simulink model "ResistiveLoad"  (R2019a)
settings: Solver=VariableStepAuto  StartTime=0.0  StopTime=2  RelTol=1e-3
libraries: powerlib x16, powerlib_meascontrol x2, simulink x1
settings Model: Creator=hakan  LastModifiedBy=hakan

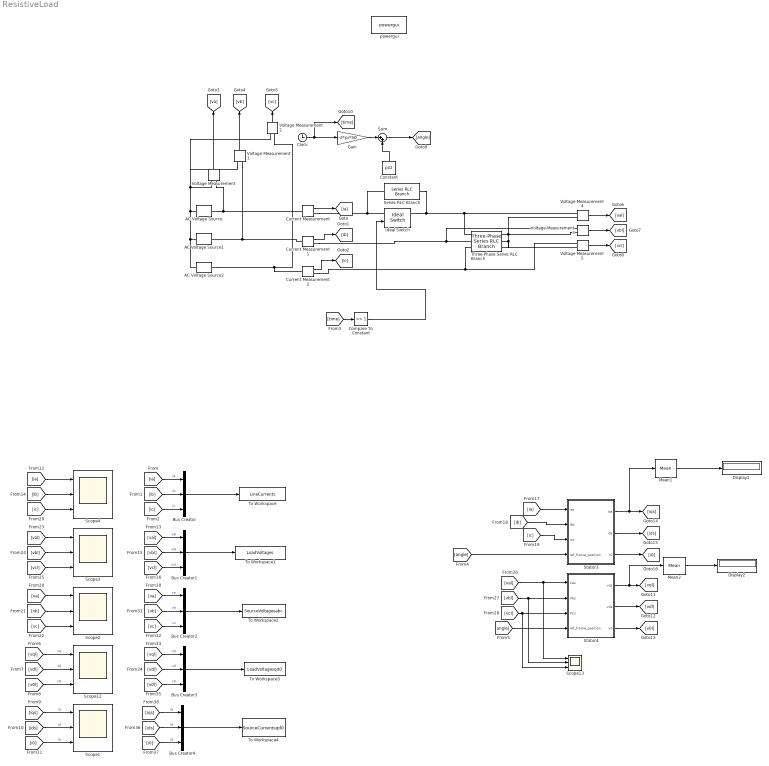
== system ResistiveLoad ==
  AC Voltage Source : powerlib/Electrical Sources/AC Voltage Source  Amplitude=400  Phase=0  Frequency=50  SampleTime=0  Measurements=None  BusType=swing  Pref=10e3  Qref=0  Qmin=-inf  Qmax=+inf
      settings: SourceProductName=Simscape Electrical
  AC Voltage Source1 : powerlib/Electrical Sources/AC Voltage Source  Amplitude=400  Phase=120  Frequency=50  SampleTime=0  Measurements=None  BusType=swing  Pref=10e3  Qref=0  Qmin=-inf  Qmax=+inf
      settings: SourceProductName=Simscape Electrical
  AC Voltage Source2 : powerlib/Electrical Sources/AC Voltage Source  Amplitude=400  Phase=240  Frequency=50  SampleTime=0  Measurements=None  BusType=swing  Pref=10e3  Qref=0  Qmin=-inf  Qmax=+inf
      settings: SourceProductName=Simscape Electrical
  Bus Creator{,1..4} (5 alike) : BusCreator  Inputs=3
  Clock : Clock
  Compare To Constant : simulink/Logic and Bit Operations/Compare To Constant  relop=<=  const=1  OutDataTypeStr=boolean
  Constant : Constant  Value=pi/2
  Current Measurement : powerlib/Measurements/Current Measurement  PhasorSimulation=off  OutputType=Complex  PSBequivalent=0
      settings: SourceProductName=Simscape Electrical
  Current Measurement1 : powerlib/Measurements/Current Measurement  PhasorSimulation=off  OutputType=Complex  PSBequivalent=0
      settings: SourceProductName=Simscape Electrical
  Current Measurement2 : powerlib/Measurements/Current Measurement  PhasorSimulation=off  OutputType=Complex  PSBequivalent=0
      settings: SourceProductName=Simscape Electrical
  Display1 : Display
      settings: Decimation=5
  Display2 : Display
      settings: Decimation=5
  Gain : Gain  Gain=-2*pi*50
  Ideal Switch : powerlib/Power Electronics/Ideal Switch  Ron=0.001  Lon=0  IC=0  Rs=1e5  Cs=inf  Measurements=on
      settings: SourceProductName=Simscape Electrical
  Mean1 : powerlib_meascontrol/Measurements/Mean  Freq=25  Vinit=0  Ts=0
      settings: SourceProductName=Simscape Electrical
  Mean2 : powerlib_meascontrol/Measurements/Mean  Freq=25  Vinit=0  Ts=0
      settings: SourceProductName=Simscape Electrical
  Scope{1..4,12..13} (6 alike) : Scope  NumInputPorts=3
  Series RLC Branch : powerlib/Elements/Series RLC Branch  LConnTagsString=__new0  RConnTagsString=__new0  BranchType=R  Resistance=500000000000  Inductance=1e-3  SetiL0=off  InitialCurrent=0  Capacitance=1e-6  Setx0=off  InitialVoltage=0  Measurements=None
      settings: SourceProductName=Simscape Electrical
  Stator3 : MATLAB Function  TreatAsAtomicUnit=on
  Stator4 : MATLAB Function  TreatAsAtomicUnit=on
  Sum : Sum  Inputs=|++
  Three-Phase Series RLC Branch : powerlib/Elements/Three-Phase Series RLC Branch  LConnTagsString=A|B|C  RConnTagsString=A|B|C  BranchType=R  Resistance=1  Inductance=1e-3  Capacitance=1e-6  Measurements=None
      settings: SourceProductName=Simscape Electrical
  To Workspace : ToWorkspace  VariableName=LineCurrents  SaveFormat=Timeseries  SampleTime=-1
  To Workspace1 : ToWorkspace  VariableName=LoadVoltages  SaveFormat=Timeseries  SampleTime=-1
  To Workspace2 : ToWorkspace  VariableName=SourceVoltagesabc  SaveFormat=Timeseries  SampleTime=-1
  To Workspace3 : ToWorkspace  VariableName=LoadVoltagesqd0  SaveFormat=Timeseries  SampleTime=-1
  To Workspace4 : ToWorkspace  VariableName=SourceCurrentsqd0  SaveFormat=Timeseries  SampleTime=-1
  Voltage Measurement{,1..5} (6 alike) : powerlib/Measurements/Voltage Measurement  PhasorSimulation=off  OutputType=Complex  PSBequivalent=0
      settings: SourceProductName=Simscape Electrical
  powergui : powerlib/powergui  Priority=1  SimulationMode=Discrete  SampleTime=10e-6  frequency=60  Iterations=50  frequencyindice=50  Pbase=100e6  ErrMax=1e-4  UnitsV=kV  UnitsW=MW  buscounter=0  FunctionMessages=off  echomessages=off  EnableUseOfTLC=off  CurrentSourceSwitches=off  DisableSnubberDevices=off  DisableRonSwitches=off  DisableVfSwitches=off  DisplayEquations=off  AutomaticDiscreteSolvers=off  SolverType=Tustin/Backward Euler (TBE)  Interpol=off  ExternalGateDelay=off  methode=off  Ts=100  x0status=blocks  SPID=on  SwTol=0  HookPort=off  NonlinearTolerance=0  nMaxIteration=15  ContinueOnMaxIteration=off  RestoreLinks=warning  ResistiveCurrentMeasurement=off  Frange=[0:2:500]  Ylog=off  Xlog=on  ShowGrid=off  save=off  variable=ZData  structure=0  ZoomFFT=off  StartTime=0.0  cycles=1  DisplayStyle=1  fundamental=60  FreqAxis=off  MaxFrequency=1000  frequencyindicesteady=1  RmsSteady=1  display=off
      settings: SourceProductName=Simscape Electrical
  wires:
  Clock/1 -> [time], Gain/1
  Compare To Constant/1 -> Ideal Switch/1
  Current Measurement/1 -> [ia]
  Current Measurement1/1 -> [ib]
  Current Measurement2/1 -> [ic]
  [ia] -> Bus Creator/1  "ia"
  [ib] -> Bus Creator/2  "ib"
  [ic] -> Bus Creator/3  "ic"
  Voltage Measurement2/1 -> [vc]
  Voltage Measurement1/1 -> [vb]
  Voltage Measurement/1 -> [va]
  Gain/1 -> Sum/1
  Constant/1 -> Sum/2
  Stator3/1(iqs) -> [iqs], Mean1/1
  [ib] -> Stator3/2(ibs)
  [ia] -> Stator3/1(ias)
  [ic] -> Stator3/3(ics)
  Mean1/1 -> Display1/1
  [va] -> Scope2/1
  [vb] -> Scope2/2
  [vc] -> Scope2/3
  Voltage Measurement4/1 -> [val]
  Voltage Measurement3/1 -> [vbl]
  Voltage Measurement5/1 -> [vcl]
  [vcl] -> Scope13/3, Stator4/3(Vcs)
  [val] -> Scope13/1, Stator4/1(Vas)
  [vbl] -> Scope13/2, Stator4/2(Vbs)
  Stator4/1(vqs) -> [vql], Mean2/1
  Mean2/1 -> Display2/1
  Sum/1 -> [angle]
  [time] -> Compare To Constant/1
  [angle] -> Stator3/4(ref_frame_position)
  [angle] -> Stator4/4(ref_frame_position)
  Stator4/3(v0) -> [v0l]
  Stator4/2(vds) -> [vdl]
  Stator3/2(ids) -> [ids]
  Stator3/3(i0) -> [i0]
  [vql] -> Scope12/1  "vq"
  [vdl] -> Scope12/2  "vd"
  [v0l] -> Scope12/3  "v0"
  [iqs] -> Scope1/1  "iq"
  [ids] -> Scope1/2  "id"
  [i0] -> Scope1/3  "i0"
  [val] -> Scope3/1
  [vbl] -> Scope3/2
  [vcl] -> Scope3/3
  [ib] -> Scope4/2
  [ia] -> Scope4/1
  [ic] -> Scope4/3
  Bus Creator/1 -> To Workspace/1
  Bus Creator1/1 -> To Workspace1/1
  Bus Creator2/1 -> To Workspace2/1
  Bus Creator3/1 -> To Workspace3/1
  Bus Creator4/1 -> To Workspace4/1
  [vcl] -> Bus Creator1/3  "vcl"
  [vbl] -> Bus Creator1/2  "vbl"
  [val] -> Bus Creator1/1  "val"
  [vc] -> Bus Creator2/3  "vc"
  [vb] -> Bus Creator2/2  "vb"
  [va] -> Bus Creator2/1  "va"
  [v0l] -> Bus Creator3/3  "v0"
  [vdl] -> Bus Creator3/2  "vd"
  [vql] -> Bus Creator3/1  "vq"
  [i0] -> Bus Creator4/3  "i0"
  [iqs] -> Bus Creator4/1  "iq"
  [ids] -> Bus Creator4/2  "id"
  connections:
  AC Voltage Source/LConn1 -- Voltage Measurement2/LConn2 -- Voltage Measurement1/LConn2 -- Voltage Measurement/LConn2 -- AC Voltage Source2/LConn1 -- AC Voltage Source1/LConn1
  AC Voltage Source/RConn1 -- Voltage Measurement/LConn1 -- Current Measurement/LConn1
  Current Measurement/RConn1 -- Ideal Switch/LConn1 -- Series RLC Branch/LConn1
  Current Measurement1/LConn1 -- Voltage Measurement1/LConn1 -- AC Voltage Source1/RConn1
  Current Measurement1/RConn1 -- Three-Phase Series RLC Branch/LConn2 -- Voltage Measurement3/LConn1
  AC Voltage Source2/RConn1 -- Voltage Measurement2/LConn1 -- Current Measurement2/LConn1
  Current Measurement2/RConn1 -- Voltage Measurement5/LConn1 -- Three-Phase Series RLC Branch/LConn3
  Series RLC Branch/RConn1 -- Voltage Measurement4/LConn1 -- Three-Phase Series RLC Branch/LConn1 -- Ideal Switch/RConn1
  Voltage Measurement4/LConn2 -- Voltage Measurement3/LConn2 -- Three-Phase Series RLC Branch/RConn3 -- Voltage Measurement5/LConn2 -- Three-Phase Series RLC Branch/RConn2 -- Three-Phase Series RLC Branch/RConn1

== matlab function ResistiveLoad/Stator3 ==
  data: iqs output; ids output; ias input; ibs input; ics input; ref_frame_position input; i0 output
function [iqs,ids,i0 ]  = fcn(ias,ibs,ics,ref_frame_position)





ids = 2/3*(ias*sin(ref_frame_position)+ibs*sin(ref_frame_position-2*pi/3)+ics*sin(ref_frame_position+2*pi/3));
iqs =  2/3*(ias*cos(ref_frame_position)+ibs*cos(ref_frame_position-2*pi/3)+ics*cos(ref_frame_position+2*pi/3));
i0 = 2/3*1/2*(ias+ibs+ics);
% iqs = (vqs-fluxlinkage_qs_derivative-ref_frame_velocity*fluxlinkage_ds)/rs;
% ids = (vds-fluxlinkage_ds_derivative+ref_frame_velocity*fluxlinkage_qs)/rs;

== matlab function ResistiveLoad/Stator4 ==
  data: vqs output; vds output; Vas input; Vbs input; Vcs input; ref_frame_position input; v0 output
function [vqs,vds,v0 ]  = fcn(Vas,Vbs,Vcs,ref_frame_position)





vds = 2/3*(Vas*sin(ref_frame_position)+Vbs*sin(ref_frame_position-2*pi/3)+Vcs*sin(ref_frame_position+2*pi/3));
vqs =  2/3*(Vas*cos(ref_frame_position)+Vbs*cos(ref_frame_position-2*pi/3)+Vcs*cos(ref_frame_position+2*pi/3));
v0 = 2/3*1/2*(Vas+Vbs+Vcs);
% iqs = (vqs-fluxlinkage_qs_derivative-ref_frame_velocity*fluxlinkage_ds)/rs;
% ids = (vds-fluxlinkage_ds_derivative+ref_frame_velocity*fluxlinkage_qs)/rs;
